simulink model "Excavator_Motion_B3D"  (R2026a)
settings: Solver=ode3  StopTime=activeTestPos.getElement('swingAng').Time(end)  FixedStep=Ts_DEM  MaxStep=0.1  AbsTol=1e-3
PostLoadFcn:
  | set_param(bdroot,'IgnoredZcDiagnostic','none');
  | activeTestPos = ScenarioMotion.Dig;
  | activeScenario = 'Dig';
  | bucketLoadsActive = 1;
model workspace: external: MAT-File ExcavatorAssemblyDataStruct.mat (data not in the file)
undefined symbols (not defined in the file or in its folder): Bo, boxHeight, boxInnerSurfaceLength, boxInnerSurfaceWidth, boxThickness, Bu, gravity, materialWeight, P28Assembly, startDiggingZPos, velocityToYForceGain, X, Y, yForceMax, yForceToZForceGain, Z, zForceMax
libraries: sm_lib x90, nesl_utility x53, Excavator_Parts_Lib x8, simulink x2, B3D_lib x1, simulink_extras x1
(part 4 of 4)

== system Excavator_Motion_B3D/Excavator/Machine/Bucket Cyl/BucketPiston ==
  BucketPiston_primary : sm_lib/Body Elements/File Solid  ExtGeomFileName=BucketPiston_Primary.SLDPRT  UnitType=FromFile  ExtGeomFileUnits=m  StepReaderType=HEX  ExportConvexHullGeometry=off  InertiaType=Custom  BasedOnType=DensityFromFile  Density=1000  DensityUnits=kg/m^3  Mass=P28Assembly.bodyGroups(11).subGroups(1).inertialProperties.mass  MassUnits=kg  CenterOfMass=P28Assembly.bodyGroups(11).subGroups(1).inertialProperties.centerOfMass  CenterOfMassUnits=m  MomentsOfInertia=P28Assembly.bodyGroups(11).subGroups(1).inertialProperties.momentsOfInertia  MomentsOfInertiaUnits=kg*m^2  ProductsOfInertia=P28Assembly.bodyGroups(11).subGroups(1).inertialProperties.productsOfInertia  ProductsOfInertiaUnits=kg*m^2  GraphicType=FromGeometry  MarkerShape=Sphere  MarkerSize=10  GraphicVisPropType=SimpleVisualProperties  GraphicDiffuseColor=P28Assembly.bodyGroups(11).subGroups(1).visualProperties.rgb  GraphicOpacity=P28Assembly.bodyGroups(11).subGroups(1).visualProperties.opacity  GraphicSpecularColor=[0.5 0.5 0.5 1.0]  GraphicAmbientColor=[0.15 0.15 0.15 1.0]  GraphicEmissiveColor=[0.0 0.0 0.0 1.0]  GraphicShininess=75  DoExposeReferenceFrame=on  SerializedFrames=<Frames/>
  RT_BucketCylToBucketPiston : sm_lib/Frames and Transforms/Rigid Transform  RotationMethod=RotationMatrix  FollAlignAxisA=+X  BaseAlignAxisA=+Y  FollAlignAxisB=+Y  BaseAlignAxisB=+Z  RotationStandardAxis=+Z  RotationAngle=0.0  RotationAngleUnits=deg  RotationArbitraryAxis=[0 0 1]  RotationSequenceAxes=FollowerAxes  RotationSequence=XYX  RotationSequenceAngles=[0 0 0]  RotationSequenceAnglesUnits=deg  RotationMatrix=P28Assembly.coordSys(21).transform.rotation  Quaternion=[1 0 0 0]  TranslationMethod=Cartesian  TranslationCartesianOffset=P28Assembly.coordSys(21).transform.translation  TranslationCartesianOffsetUnits=m  TranslationStandardAxis=+Z  TranslationStandardOffset=0  TranslationStandardOffsetUnits=m  TranslationROffset=0  TranslationROffsetUnits=m  TranslationThetaOffset=0  TranslationThetaOffsetUnits=deg  TranslationZOffset=0  TranslationZOffsetUnits=m
  RT_BucketPistonToBucketLink : sm_lib/Frames and Transforms/Rigid Transform  RotationMethod=RotationMatrix  FollAlignAxisA=+X  BaseAlignAxisA=+Y  FollAlignAxisB=+Y  BaseAlignAxisB=+Z  RotationStandardAxis=+Z  RotationAngle=0.0  RotationAngleUnits=deg  RotationArbitraryAxis=[0 0 1]  RotationSequenceAxes=FollowerAxes  RotationSequence=XYX  RotationSequenceAngles=[0 0 0]  RotationSequenceAnglesUnits=deg  RotationMatrix=P28Assembly.coordSys(12).transform.rotation  Quaternion=[1 0 0 0]  TranslationMethod=Cartesian  TranslationCartesianOffset=P28Assembly.coordSys(12).transform.translation  TranslationCartesianOffsetUnits=m  TranslationStandardAxis=+Z  TranslationStandardOffset=0  TranslationStandardOffsetUnits=m  TranslationROffset=0  TranslationROffsetUnits=m  TranslationThetaOffset=0  TranslationThetaOffsetUnits=deg  TranslationZOffset=0  TranslationZOffsetUnits=m
  B1 : PMIOPort  Side=Left
  F1 : PMIOPort  Port=2  Side=Right
  connections:
  BucketPiston_primary/RConn1 -- RT_BucketCylToBucketPiston/LConn1 -- RT_BucketPistonToBucketLink/LConn1
  RT_BucketCylToBucketPiston/RConn1 -- B1/RConn1
  RT_BucketPistonToBucketLink/RConn1 -- F1/RConn1

== system Excavator_Motion_B3D/Excavator/Machine/BucketLoads/BucketLoadsVariant ==
  BucketAngle : Inport
  BucketLoadsActive : Subsystem  VariantControl=bucketLoadsActive==true
  BucketLoadsInactive : Subsystem  VariantControl=bucketLoadsActive==false
  BucketCOM : PMIOPort  Side=Left
  BucketForceY : Outport
  BucketForceZ : Outport  Port=2

== system Excavator_Motion_B3D/Excavator/Machine/Stick Cyl/StickCyl ==
  RT_BoomToStickCyl : sm_lib/Frames and Transforms/Rigid Transform  RotationMethod=RotationMatrix  FollAlignAxisA=+X  BaseAlignAxisA=+Y  FollAlignAxisB=+Y  BaseAlignAxisB=+Z  RotationStandardAxis=+Z  RotationAngle=0.0  RotationAngleUnits=deg  RotationArbitraryAxis=[0 0 1]  RotationSequenceAxes=FollowerAxes  RotationSequence=XYX  RotationSequenceAngles=[0 0 0]  RotationSequenceAnglesUnits=deg  RotationMatrix=P28Assembly.coordSys(9).transform.rotation  Quaternion=[1 0 0 0]  TranslationMethod=Cartesian  TranslationCartesianOffset=P28Assembly.coordSys(9).transform.translation  TranslationCartesianOffsetUnits=m  TranslationStandardAxis=+Z  TranslationStandardOffset=0  TranslationStandardOffsetUnits=m  TranslationROffset=0  TranslationROffsetUnits=m  TranslationThetaOffset=0  TranslationThetaOffsetUnits=deg  TranslationZOffset=0  TranslationZOffsetUnits=m
  RT_StickCylToStickPiston : sm_lib/Frames and Transforms/Rigid Transform  RotationMethod=RotationMatrix  FollAlignAxisA=+X  BaseAlignAxisA=+Y  FollAlignAxisB=+Y  BaseAlignAxisB=+Z  RotationStandardAxis=+Z  RotationAngle=0.0  RotationAngleUnits=deg  RotationArbitraryAxis=[0 0 1]  RotationSequenceAxes=FollowerAxes  RotationSequence=XYX  RotationSequenceAngles=[0 0 0]  RotationSequenceAnglesUnits=deg  RotationMatrix=P28Assembly.coordSys(20).transform.rotation  Quaternion=[1 0 0 0]  TranslationMethod=Cartesian  TranslationCartesianOffset=P28Assembly.coordSys(20).transform.translation  TranslationCartesianOffsetUnits=m  TranslationStandardAxis=+Z  TranslationStandardOffset=0  TranslationStandardOffsetUnits=m  TranslationROffset=0  TranslationROffsetUnits=m  TranslationThetaOffset=0  TranslationThetaOffsetUnits=deg  TranslationZOffset=0  TranslationZOffsetUnits=m
  StickCyl_primary : sm_lib/Body Elements/File Solid  ExtGeomFileName=StickCyl_Primary.SLDPRT  UnitType=FromFile  ExtGeomFileUnits=m  StepReaderType=HEX  ExportConvexHullGeometry=off  InertiaType=Custom  BasedOnType=DensityFromFile  Density=1000  DensityUnits=kg/m^3  Mass=P28Assembly.bodyGroups(8).subGroups(1).inertialProperties.mass  MassUnits=kg  CenterOfMass=P28Assembly.bodyGroups(8).subGroups(1).inertialProperties.centerOfMass  CenterOfMassUnits=m  MomentsOfInertia=P28Assembly.bodyGroups(8).subGroups(1).inertialProperties.momentsOfInertia  MomentsOfInertiaUnits=kg*m^2  ProductsOfInertia=P28Assembly.bodyGroups(8).subGroups(1).inertialProperties.productsOfInertia  ProductsOfInertiaUnits=kg*m^2  GraphicType=FromGeometry  MarkerShape=Sphere  MarkerSize=10  GraphicVisPropType=SimpleVisualProperties  GraphicDiffuseColor=P28Assembly.bodyGroups(8).subGroups(1).visualProperties.rgb  GraphicOpacity=P28Assembly.bodyGroups(8).subGroups(1).visualProperties.opacity  GraphicSpecularColor=[0.5 0.5 0.5 1.0]  GraphicAmbientColor=[0.15 0.15 0.15 1.0]  GraphicEmissiveColor=[0.0 0.0 0.0 1.0]  GraphicShininess=75  DoExposeReferenceFrame=on  SerializedFrames=<Frames/>
  B1 : PMIOPort  Side=Left
  F1 : PMIOPort  Port=2  Side=Right
  connections:
  RT_BoomToStickCyl/LConn1 -- StickCyl_primary/RConn1 -- RT_StickCylToStickPiston/LConn1
  RT_BoomToStickCyl/RConn1 -- B1/RConn1
  RT_StickCylToStickPiston/RConn1 -- F1/RConn1

== system Excavator_Motion_B3D/Excavator/Machine/Stick Cyl/StickCylToStickPiston ==
  PS-Simulink Converter : nesl_utility/PS-Simulink Converter  PhysicalDomain=network_engine_domain  SubClassName=ps_output  LeftPortType=input  RightPortType=output  PseudoPeriodic=off  Frequencies=[]  VectorFormat=inherit  Unit=inherit  AffineConversion=off
  PS-Simulink Converter1 : nesl_utility/PS-Simulink Converter  PhysicalDomain=network_engine_domain  SubClassName=ps_output  LeftPortType=input  RightPortType=output  PseudoPeriodic=off  Frequencies=[]  VectorFormat=inherit  Unit=inherit  AffineConversion=off
  StickCylToStickPiston : sm_lib/Joints/Cylindrical Joint  JointMode=Normal  CompositeWrenchDir=FollowerOnBase  CompositeWrenchFrame=BaseFrame  SenseConstraintForce=off  SenseConstraintTorque=off  SenseTotalForce=off  SenseTotalTorque=off  RzPositionTargetSpecify=off  RzPositionTargetPriority=High  RzPositionTargetValue=0  RzPositionTargetValueUnits=deg  RzVelocityTargetSpecify=off  RzVelocityTargetPriority=High  RzVelocityTargetValue=0  RzVelocityTargetValueUnits=deg/s  RzEquilibriumPosition=0  RzEquilibriumPositionUnits=deg  RzSpringStiffness=0  RzSpringStiffnessUnits=N*m/deg  RzDampingCoefficient=0  RzDampingCoefficientUnits=N*m/(deg/s)  RzLowerLimitSpecify=off  RzLowerLimitBound=-90  RzLowerLimitBoundUnits=deg  RzLowerLimitStiffness=1e4  RzLowerLimitStiffnessUnits=N*m/deg  RzLowerLimitDamping=10  RzLowerLimitDampingUnits=N*m/(deg/s)  RzLowerLimitTransitionRegionWidth=0.1  RzLowerLimitTransitionRegionWidthUnits=deg  RzUpperLimitSpecify=off  RzUpperLimitBound=90  RzUpperLimitBoundUnits=deg  RzUpperLimitStiffness=1e4  RzUpperLimitStiffnessUnits=N*m/deg  RzUpperLimitDamping=10  RzUpperLimitDampingUnits=N*m/(deg/s)  RzUpperLimitTransitionRegionWidth=0.1  RzUpperLimitTransitionRegionWidthUnits=deg  RzTorqueActuationMode=NoTorque  RzMotionActuationMode=ComputedMotion  RzSensePosition=off  RzSenseVelocity=off  RzSenseAcceleration=off  RzSenseTorqueForce=off  RzSenseLowerLimitTorqueForce=off  RzSenseUpperLimitTorqueForce=off  PzPositionTargetSpecify=on  PzPositionTargetPriority=High  PzPositionTargetValue=activeTestPos.getElement('stickPos').Data(1)  PzPositionTargetValueUnits=mm  PzVelocityTargetSpecify=off  PzVelocityTargetPriority=High  PzVelocityTargetValue=0  PzVelocityTargetValueUnits=m/s  PzEquilibriumPosition=0  PzEquilibriumPositionUnits=m  PzSpringStiffness=0  PzSpringStiffnessUnits=N/m  PzDampingCoefficient=0  PzDampingCoefficientUnits=N/(m/s)  PzLowerLimitSpecify=off  PzLowerLimitBound=-1  PzLowerLimitBoundUnits=m  PzLowerLimitStiffness=1e6  PzLowerLimitStiffnessUnits=N/m  PzLowerLimitDamping=1e3  PzLowerLimitDampingUnits=N/(m/s)  PzLowerLimitTransitionRegionWidth=1e-4  PzLowerLimitTransitionRegionWidthUnits=m  PzUpperLimitSpecify=off  PzUpperLimitBound=1  PzUpperLimitBoundUnits=m  PzUpperLimitStiffness=1e6  PzUpperLimitStiffnessUnits=N/m  PzUpperLimitDamping=1e3  PzUpperLimitDampingUnits=N/(m/s)  PzUpperLimitTransitionRegionWidth=1e-4  PzUpperLimitTransitionRegionWidthUnits=m  PzTorqueActuationMode=ComputedTorque  PzMotionActuationMode=InputMotion  PzSensePosition=on  PzSenseVelocity=off  PzSenseAcceleration=off  PzSenseTorqueForce=on  PzSenseLowerLimitTorqueForce=off  PzSenseUpperLimitTorqueForce=off
  B : PMIOPort  Side=Left
  F : PMIOPort  Port=2  Side=Right
  pz : PMIOPort  Port=3  Side=Left
  Out Bus Element : Outport  PortName=m  Element=p
  Out Bus Element1 : Outport  PortName=m  Element=frc
  wires:
  PS-Simulink Converter1/1 -> Out Bus Element1/1
  PS-Simulink Converter/1 -> Out Bus Element/1
  connections:
  B/RConn1 -- StickCylToStickPiston/LConn1
  StickCylToStickPiston/RConn1 -- F/RConn1
  pz/RConn1 -- StickCylToStickPiston/LConn2
  StickCylToStickPiston/RConn3 -- PS-Simulink Converter1/LConn1
  StickCylToStickPiston/RConn2 -- PS-Simulink Converter/LConn1

== system Excavator_Motion_B3D/Excavator/Machine/Stick Cyl/StickPiston ==
  RT_StickCylToStickPiston : sm_lib/Frames and Transforms/Rigid Transform  RotationMethod=RotationMatrix  FollAlignAxisA=+X  BaseAlignAxisA=+Y  FollAlignAxisB=+Y  BaseAlignAxisB=+Z  RotationStandardAxis=+Z  RotationAngle=0.0  RotationAngleUnits=deg  RotationArbitraryAxis=[0 0 1]  RotationSequenceAxes=FollowerAxes  RotationSequence=XYX  RotationSequenceAngles=[0 0 0]  RotationSequenceAnglesUnits=deg  RotationMatrix=P28Assembly.coordSys(20).transform.rotation  Quaternion=[1 0 0 0]  TranslationMethod=Cartesian  TranslationCartesianOffset=P28Assembly.coordSys(20).transform.translation  TranslationCartesianOffsetUnits=m  TranslationStandardAxis=+Z  TranslationStandardOffset=0  TranslationStandardOffsetUnits=m  TranslationROffset=0  TranslationROffsetUnits=m  TranslationThetaOffset=0  TranslationThetaOffsetUnits=deg  TranslationZOffset=0  TranslationZOffsetUnits=m
  RT_StickPistonToStick : sm_lib/Frames and Transforms/Rigid Transform  RotationMethod=RotationMatrix  FollAlignAxisA=+X  BaseAlignAxisA=+Y  FollAlignAxisB=+Y  BaseAlignAxisB=+Z  RotationStandardAxis=+Z  RotationAngle=0.0  RotationAngleUnits=deg  RotationArbitraryAxis=[0 0 1]  RotationSequenceAxes=FollowerAxes  RotationSequence=XYX  RotationSequenceAngles=[0 0 0]  RotationSequenceAnglesUnits=deg  RotationMatrix=P28Assembly.coordSys(10).transform.rotation  Quaternion=[1 0 0 0]  TranslationMethod=Cartesian  TranslationCartesianOffset=P28Assembly.coordSys(10).transform.translation  TranslationCartesianOffsetUnits=m  TranslationStandardAxis=+Z  TranslationStandardOffset=0  TranslationStandardOffsetUnits=m  TranslationROffset=0  TranslationROffsetUnits=m  TranslationThetaOffset=0  TranslationThetaOffsetUnits=deg  TranslationZOffset=0  TranslationZOffsetUnits=m
  StickPiston_primary : sm_lib/Body Elements/File Solid  ExtGeomFileName=StickPiston_Primary.SLDPRT  UnitType=FromFile  ExtGeomFileUnits=m  StepReaderType=HEX  ExportConvexHullGeometry=off  InertiaType=Custom  BasedOnType=DensityFromFile  Density=1000  DensityUnits=kg/m^3  Mass=P28Assembly.bodyGroups(9).subGroups(1).inertialProperties.mass  MassUnits=kg  CenterOfMass=P28Assembly.bodyGroups(9).subGroups(1).inertialProperties.centerOfMass  CenterOfMassUnits=m  MomentsOfInertia=P28Assembly.bodyGroups(9).subGroups(1).inertialProperties.momentsOfInertia  MomentsOfInertiaUnits=kg*m^2  ProductsOfInertia=P28Assembly.bodyGroups(9).subGroups(1).inertialProperties.productsOfInertia  ProductsOfInertiaUnits=kg*m^2  GraphicType=FromGeometry  MarkerShape=Sphere  MarkerSize=10  GraphicVisPropType=SimpleVisualProperties  GraphicDiffuseColor=P28Assembly.bodyGroups(9).subGroups(1).visualProperties.rgb  GraphicOpacity=P28Assembly.bodyGroups(9).subGroups(1).visualProperties.opacity  GraphicSpecularColor=[0.5 0.5 0.5 1.0]  GraphicAmbientColor=[0.15 0.15 0.15 1.0]  GraphicEmissiveColor=[0.0 0.0 0.0 1.0]  GraphicShininess=75  DoExposeReferenceFrame=on  SerializedFrames=<Frames/>
  B1 : PMIOPort  Side=Right
  B2 : PMIOPort  Port=2  Side=Left
  connections:
  RT_StickPistonToStick/LConn1 -- StickPiston_primary/RConn1 -- RT_StickCylToStickPiston/LConn1
  RT_StickPistonToStick/RConn1 -- B1/RConn1
  RT_StickCylToStickPiston/RConn1 -- B2/RConn1

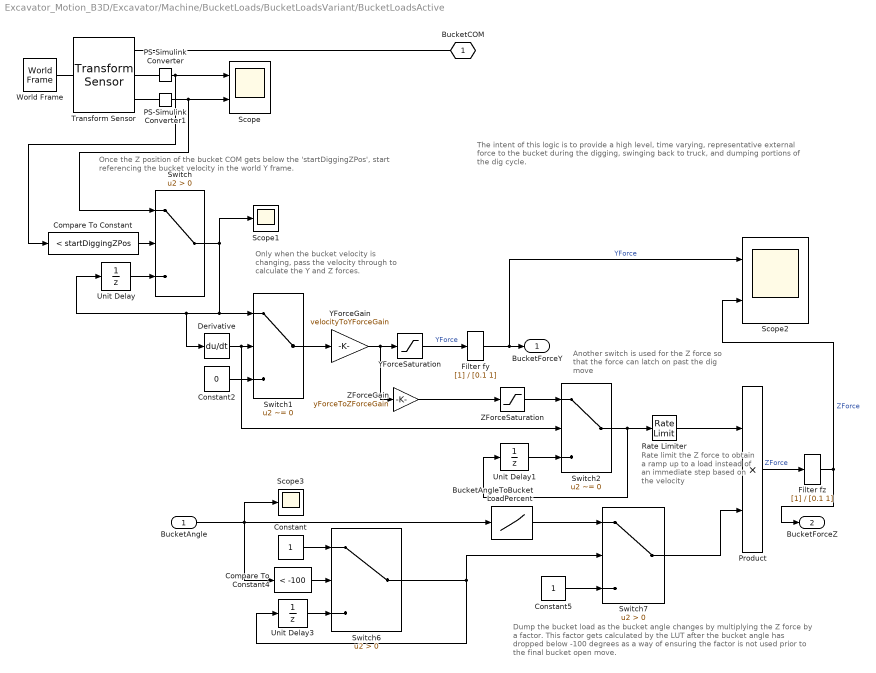
== system Excavator_Motion_B3D/Excavator/Machine/BucketLoads/BucketLoadsVariant/BucketLoadsActive ==
  note: Once the Z position of the bucket COM gets below the 'startDiggingZPos', start referencing the bucket velocity in the world Y frame.
  note: Only when the bucket velocity is changing, pass the velocity through to calculate the Y and Z forces.
  note: Dump the bucket load as the bucket angle changes by multiplying the Z force by a factor. This factor gets calculated by the LUT after the bucket angle has dropped below -100 degrees as a way of ensuring the factor is not used prior to the final bucket open move.
  note: Another switch is used for the Z force so that the force can latch on past the dig move
  note: Rate limit the Z force to obtain a ramp up to a load instead of an immediate step based on the velocity
  note: The intent of this logic is to provide a high level, time varying, representative external force to the bucket during the digging, swinging back to truck, and dumping portions of the dig cycle.
  BucketAngle : Inport
  BucketAngleToBucketLoadPercent : Lookup_n-D  NumberOfTableDimensions=1  BreakpointsForDimension1=[-100 -20]  Table=[1 0]  ExtrapMethod=Clip  UseLastTableValue=on  InternalRulePriority=Speed  RndMeth=Simplest
  Compare To Constant : simulink/Logic and Bit Operations/Compare To Constant  relop=<  const=startDiggingZPos  OutDataTypeStr=boolean
  Compare To Constant4 : simulink/Logic and Bit Operations/Compare To Constant  relop=<  const=-100  OutDataTypeStr=boolean
  Constant : Constant
  Constant2 : Constant  Value=0
  Constant5 : Constant
  Derivative : Derivative
  Filter fy : TransferFcn  Denominator=[0.1 1]
  Filter fz : TransferFcn  Denominator=[0.1 1]
  PS-Simulink Converter : nesl_utility/PS-Simulink Converter  PhysicalDomain=network_engine_domain  SubClassName=ps_output  LeftPortType=input  RightPortType=output  PseudoPeriodic=off  Frequencies=[]  VectorFormat=inherit  Unit=mm  AffineConversion=off
  PS-Simulink Converter1 : nesl_utility/PS-Simulink Converter  PhysicalDomain=network_engine_domain  SubClassName=ps_output  LeftPortType=input  RightPortType=output  PseudoPeriodic=off  Frequencies=[]  VectorFormat=inherit  Unit=mm/s  AffineConversion=off
  Product : Product
  Rate Limiter : RateLimiter  RisingSlewLimit=750  FallingSlewLimit=-80  SampleTimeMode=inherited
  Scope : Scope  NumInputPorts=2
      settings: ActiveDisplayYMinimum=-4867.9057  ActiveDisplayYMaximum=4889.74505
  Scope1 : Scope
      settings: ActiveDisplayYMinimum=-30.09967  ActiveDisplayYMaximum=270.897  DataLoggingVariableName=ScopeData2
  Scope2 : Scope  NumInputPorts=2
      settings: ActiveDisplayYMinimum=-174.28167  ActiveDisplayYMaximum=248.19229  DataLoggingVariableName=ScopeData3
  Scope3 : Scope
      settings: ActiveDisplayYMinimum=-124.88832  ActiveDisplayYMaximum=6.44138  DataLoggingVariableName=ScopeData5
  Switch : Switch  Criteria=u2 > Threshold  SaturateOnIntegerOverflow=off  InputSameDT=off
  Switch1 : Switch  Criteria=u2 ~= 0  SaturateOnIntegerOverflow=off  InputSameDT=off
  Switch2 : Switch  Criteria=u2 ~= 0  SaturateOnIntegerOverflow=off  InputSameDT=off
  Switch6 : Switch  Criteria=u2 > Threshold  SaturateOnIntegerOverflow=off  InputSameDT=off
  Switch7 : Switch  Criteria=u2 > Threshold  SaturateOnIntegerOverflow=off  InputSameDT=off
  Transform Sensor : sm_lib/Frames and Transforms/Transform Sensor  MeasurementFrame=World  RotationSequence=XYX  SenseAngle=off  SenseAxis=off  SenseQ=off  SenseR=off  SenseRotationSequence=off  SenseOmegaX=off  SenseOmegaY=off  SenseOmegaZ=off  SenseOmega=off  SenseQDot=off  SenseRDot=off  SenseRotationSequenceDot=off  SenseAlphaX=off  SenseAlphaY=off  SenseAlphaZ=off  SenseAlpha=off  SenseQDDot=off  SenseRDDot=off  SenseX=off  SenseY=off  SenseZ=on  SenseXYZ=off  SenseRad=off  SenseAzim=off  SenseDist=off  SenseInc=off  SenseXDot=off  SenseYDot=on  SenseZDot=off  SenseXYZDot=off  SenseRadDot=off  SenseAzimDot=off  SenseDistDot=off  SenseIncDot=off  SenseXDDot=off  SenseYDDot=off  SenseZDDot=off  SenseXYZDDot=off  SenseRadDDot=off  SenseAzimDDot=off  SenseDistDDot=off  SenseIncDDot=off
  Unit Delay : UnitDelay  SampleTime=-1
  Unit Delay1 : UnitDelay  SampleTime=-1
  Unit Delay3 : UnitDelay  SampleTime=-1
  World Frame : sm_lib/Frames and Transforms/World Frame
  YForceGain : Gain  Gain=velocityToYForceGain
  YForceSaturation : Saturate  UpperLimit=yForceMax  LowerLimit=0
  ZForceGain : Gain  Gain=yForceToZForceGain
  ZForceSaturation : Saturate  UpperLimit=-materialWeight  LowerLimit=-zForceMax
  BucketCOM : PMIOPort  Side=Left
  BucketForceY : Outport
  BucketForceZ : Outport  Port=2
  wires:
  ZForceSaturation/1 -> Switch2/1
  Unit Delay1/1 -> Switch2/3
  Filter fy/1 -> Scope2/1, BucketForceY/1  "YForce"
  Compare To Constant/1 -> Switch/2
  Unit Delay/1 -> Switch/3
  Switch1/1 -> YForceGain/1
  Switch/1 -> Switch1/1, Derivative/1, Unit Delay/1, Scope1/1
  PS-Simulink Converter/1 -> Compare To Constant/1, Scope/1
  PS-Simulink Converter1/1 -> Switch/1, Scope/2
  Constant2/1 -> Switch1/3
  Switch2/1 -> Rate Limiter/1, Unit Delay1/1
  BucketAngle/1 -> Scope3/1, Compare To Constant4/1, BucketAngleToBucketLoadPercent/1
  Rate Limiter/1 -> Product/1
  Filter fz/1 -> BucketForceZ/1, Scope2/2  "ZForce"
  ZForceGain/1 -> ZForceSaturation/1
  Derivative/1 -> Switch2/2, Switch1/2
  Compare To Constant4/1 -> Switch6/2
  Unit Delay3/1 -> Switch6/3
  Constant/1 -> Switch6/1
  Switch6/1 -> Unit Delay3/1, Switch7/2
  BucketAngleToBucketLoadPercent/1 -> Switch7/1
  Constant5/1 -> Switch7/3
  Switch7/1 -> Product/2
  YForceGain/1 -> YForceSaturation/1, ZForceGain/1
  YForceSaturation/1 -> Filter fy/1  "YForce"
  Product/1 -> Filter fz/1  "ZForce"
  connections:
  PS-Simulink Converter1/LConn1 -- Transform Sensor/RConn3
  PS-Simulink Converter/LConn1 -- Transform Sensor/RConn2
  World Frame/RConn1 -- Transform Sensor/LConn1
  BucketCOM/RConn1 -- Transform Sensor/RConn1

== system Excavator_Motion_B3D/Excavator/Machine/BucketLoads/BucketLoadsVariant/BucketLoadsInactive ==
  BucketAngle : Inport
  Constant : Constant  Value=0
  Constant1 : Constant  Value=0
  Terminator : Terminator
  BucketCOM : PMIOPort  Side=Left
  BucketForceY : Outport
  BucketForceZ : Outport  Port=2
  wires:
  Constant/1 -> BucketForceY/1
  Constant1/1 -> BucketForceZ/1
  BucketAngle/1 -> Terminator/1
